simulink model "dowd_id"  (R2020b)
settings: Solver=VariableStepAuto  StartTime=0.0  StopTime=10.0  RelTol=1e-3
values from neighbouring files (symbols this model uses):
  A = [0 0 1 0 ... (first row only)    [DCMotorODE.m]    (also in downright.m)
  B = -km * Bold / Rm*gain    [DCMotorODE.m]    (also in downright.m = -km * Bold / Rm*40)
  C = eye(2,4)    [DCMotorODE.m]    (also in downright.m)
  D = zeros(2,1)    [DCMotorODE.m]    (also in downright.m)
  h = 0.01    [downright.m]
undefined symbols (not defined in the file or in its folder): Humusoft, MF634
libraries: sldrtlib x2
settings Model: Creator=zhehanli  LastModifiedBy=zhehanli

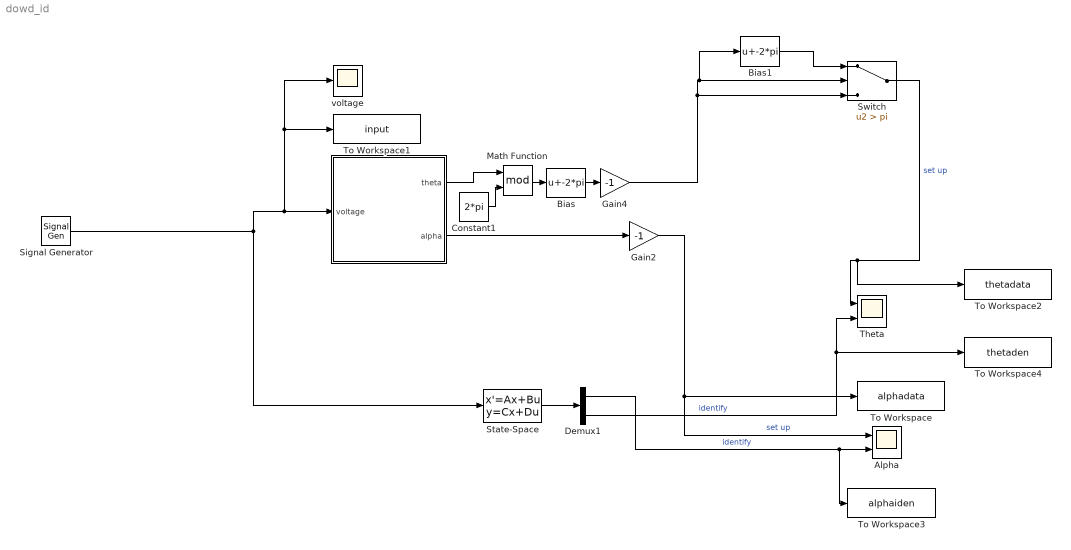
== system dowd_id ==
  "\tTheta" : Scope  NumInputPorts=2
  " " : Subsystem  LoadFcn=hwinit  InitFcn=hwinit  mask{h=h}
      mask prompts: h "Sampling period [s]"
      mask Display:
      | disp('Qube-Servo')
      | port_label('output',1,'theta')
      | port_label('output',2,'alpha')
      | port_label('input',1,'V')
  Alpha : Scope  NumInputPorts=2
  Bias : Bias  Bias=-2*pi
  Bias1 : Bias  Bias=-2*pi
  Constant1 : Constant  Value=2*pi
  Demux1 : Demux  Outputs=2
  Gain2 : Gain  Gain=-1
  Gain4 : Gain  Gain=-1
  Math Function : Math  Operator=mod  SignedPower=on  SaturateOnIntegerOverflow=on
  Signal Generator : SignalGenerator  WaveForm=random  Amplitude=0.01  Frequency=0.01
  State-Space : StateSpace  A=A  B=B  C=C  D=D  InitialCondition=[ 0 0 0 0]
  Switch : Switch  Criteria=u2 > Threshold  Threshold=pi
  To Workspace : ToWorkspace  VariableName=alphadata  SaveFormat=Timeseries  SampleTime=h
      settings: Decimation=2
  To Workspace1 : ToWorkspace  VariableName=input  SaveFormat=Timeseries  SampleTime=h
      settings: Decimation=2
  To Workspace2 : ToWorkspace  VariableName=thetadata  SaveFormat=Timeseries  SampleTime=h
      settings: Decimation=2
  To Workspace3 : ToWorkspace  VariableName=alphaiden  SaveFormat=Timeseries  SampleTime=h
      settings: Decimation=2
  To Workspace4 : ToWorkspace  VariableName=thetaden  SaveFormat=Timeseries  SampleTime=h
      settings: Decimation=2
  voltage : Scope
  wires:
  Gain4/1 -> Switch/3, Switch/2, Bias1/1
  Demux1/1 -> To Workspace3/1, Alpha/2  "identify"
  Constant1/1 -> Math Function/2
  Switch/1 -> "\tTheta"/1, To Workspace2/1  "set up"
  Bias1/1 -> Switch/1
  Signal Generator/1 -> State-Space/1, To Workspace1/1, voltage/1, " "/1(voltage)
  Math Function/1 -> Bias/1
  Demux1/2 -> "\tTheta"/2, To Workspace4/1  "identify"
  " "/1(theta) -> Math Function/1
  " "/2(alpha) -> Gain2/1
  Bias/1 -> Gain4/1
  State-Space/1 -> Demux1/1
  Gain2/1 -> To Workspace/1, Alpha/1  "set up"

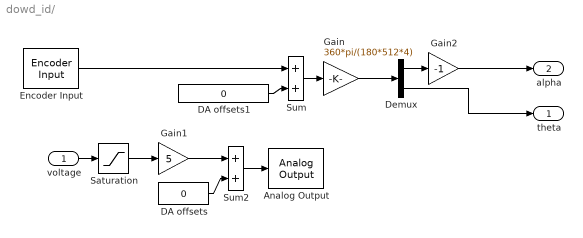
== system dowd_id/  ==
  voltage : Inport
  Analog Output : sldrtlib/Analog Output  SampleTime=h  MaxMissedTicks=100  ShowMissedTicks=off  YieldWhenWaiting=off  DrvName=Humusoft/MF634  DrvAddress=4294967295  DrvOptions=0  Channels=[1]  RangeMode=2  VoltRange=1  InitialValue=0  FinalValue=0
      settings: AttributesFormatString=Humusoft\nMF634 [auto]
  DA offsets : Constant  Value=0
  DA offsets1 : Constant  Value=0  SampleTime=h
  Demux : Demux  Outputs=2
  Encoder Input : sldrtlib/Encoder Input  SampleTime=h  MaxMissedTicks=100  ShowMissedTicks=off  YieldWhenWaiting=off  DrvName=Humusoft/MF634  DrvAddress=4294967295  DrvOptions=0  Channels=[1,2]  QuadMode=3  IndexPulse=1  InputFilter=Inf  DataType=1
      settings: AttributesFormatString=Humusoft\nMF634 [auto]
  Gain : Gain  Gain=360*pi/(180*512*4)  SaturateOnIntegerOverflow=on  OutDataTypeStr=Inherit: Same as input  ParamDataTypeStr=Inherit: Same as input
  Gain1 : Gain  Gain=5  SaturateOnIntegerOverflow=on  OutDataTypeStr=Inherit: Same as input  ParamDataTypeStr=Inherit: Same as input
  Gain2 : Gain  Gain=-1  SaturateOnIntegerOverflow=on  OutDataTypeStr=Inherit: Same as input  ParamDataTypeStr=Inherit: Same as input
  Saturation : Saturate  UpperLimit=1  LowerLimit=-1
  Sum : Sum  InputSameDT=on  SaturateOnIntegerOverflow=on  OutDataTypeStr=Inherit: Same as first input
  Sum2 : Sum  InputSameDT=on  SaturateOnIntegerOverflow=on  OutDataTypeStr=Inherit: Same as first input
  theta : Outport  Tag=Cable length
  alpha : Outport  Tag=Cable length  Port=2
  wires:
  Sum/1 -> Gain/1
  DA offsets1/1 -> Sum/2
  Gain1/1 -> Sum2/1
  Sum2/1 -> Analog Output/1
  DA offsets/1 -> Sum2/2
  voltage/1 -> Saturation/1
  Encoder Input/1 -> Sum/1
  Saturation/1 -> Gain1/1
  Demux/1 -> Gain2/1
  Gain/1 -> Demux/1
  Gain2/1 -> alpha/1
  Demux/2 -> theta/1
